simulink model "Modele_Eleve"  (R2021a)
settings: Solver=FixedStepAuto  StartTime=0.0  StopTime=10  FixedStep=2/1000  RelTol=1e-3
libraries: fl_lib x7, nesl_utility x3
settings Model: Creator=pt_ptsi  LastModifiedBy=xpess
settings SolverCC: AlgebraicLoopSolver=TrustRegion
settings DataIOCC: ReturnWorkspaceOutputs=off
settings DebuggingCC: SFMachineParentedDataDiag=warning  ArithmeticOperatorsInVariantConditions=warning
settings SFSimCC: SimUseLocalCustomCode=off  CustomCodeUndefinedFunction=UseInterfaceOnly
settings RTWCC: RTWUseLocalCustomCode=off
settings CodeAppCC: StateflowObjectComments=on
settings SimscapeCC: SimscapeNormalizeSystem=off

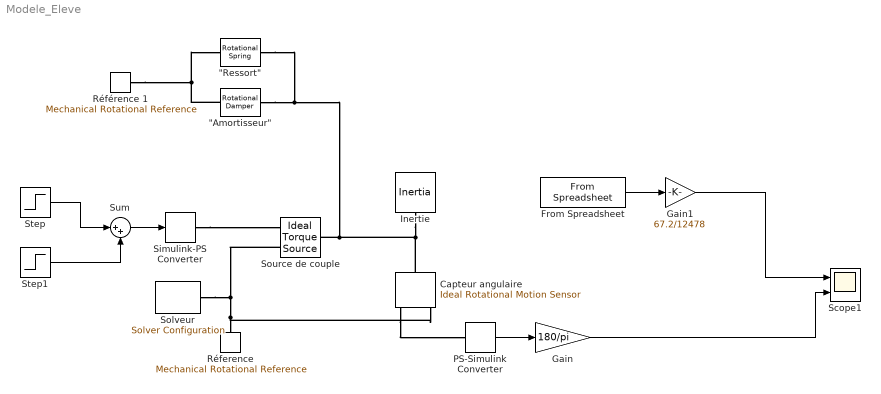
== system Modele_Eleve ==
  "\"Amortisseur\"" : fl_lib/Mechanical/Rotational Elements/Rotational Damper  D=0.01 N*m/(rad/s)  w_specify=off  w_priority=None  w=0 rad/s  w_nominal_specify=off  w_nominal_unit=rad/s  w_nominal_value=1  t_specify=off  t_priority=None  t=0 N*m  t_nominal_specify=off  t_nominal_unit=N*m  t_nominal_value=1
  "\"Ressort\"" : fl_lib/Mechanical/Rotational Elements/Rotational Spring  spr_rate=9.29 N*m/rad  w_specify=off  w_priority=None  w=0 rad/s  w_nominal_specify=off  w_nominal_unit=rad/s  w_nominal_value=1  t_specify=off  t_priority=None  t=0 N*m  t_nominal_specify=off  t_nominal_unit=N*m  t_nominal_value=1  phi_specify=off  phi_priority=High  phi=0 rad  phi_nominal_specify=off  phi_nominal_unit=rad  phi_nominal_value=1
  Capteur angulaire : fl_lib/Mechanical/Mechanical Sensors/Ideal Rotational Motion Sensor  wrap_angle=simscape.enum.onoff.off  offset=0 rad
  From Spreadsheet : FromSpreadsheet  FileName=C:\GitHub\PSI_Cy_04_ModelisationDynamique\TPs\TP_04_Drone\Essai\TestPendule.xlsx  SheetName=TestPendule  Range=A2:B502
  Gain : Gain  Gain=180/pi
  Gain1 : Gain  Gain=67.2/12478
  "Inertie " : fl_lib/Mechanical/Rotational Elements/Inertia  inertia=0.001 kg*m^2  num_ports=foundation.enum.numPorts2.one  w_specify=off  w_priority=High  w=0 rad/s  w_nominal_specify=off  w_nominal_unit=rad/s  w_nominal_value=1  t_specify=off  t_priority=None  t=0 N*m  t_nominal_specify=off  t_nominal_unit=N*m  t_nominal_value=1
  PS-Simulink Converter : nesl_utility/PS-Simulink Converter  PhysicalDomain=network_engine_domain  SubClassName=ps_output  LeftPortType=input  RightPortType=output  PseudoPeriodic=off  Frequencies=[]  Unit=1  AffineConversion=off
      settings: SourceProductBaseCode=PW,SS
  Réference : fl_lib/Mechanical/Rotational Elements/Mechanical Rotational Reference
  Référence 1 : fl_lib/Mechanical/Rotational Elements/Mechanical Rotational Reference
  Scope1 : Scope  NumInputPorts=2
  Simulink-PS Converter : nesl_utility/Simulink-PS Converter  PhysicalDomain=network_engine_domain  SubClassName=ps_input  LeftPortType=input  RightPortType=output  PseudoPeriodic=off  Frequencies=[]  NoiseDistribution=none  NoiseParameters=[]  Unit=1  AffineConversion=off  FilteringAndDerivatives=zero  SimscapeFilterOrder=1  InputFilterTimeConstant=0.001  UdotUserProvided=1
      settings: SourceProductBaseCode=PW,SS
  Solveur : nesl_utility/Solver Configuration  PhysicalDomain=network_engine_domain  SubClassName=solver  LeftPortType=input  RightPortType=generic  Tones=[]  Harmonics=[]  SimulateNoise=off  Profile=off  UseLocalSampling=off  EnableSwitchedLinearOptims=on  FrequencyDomain=off  UseCCode=off  RelTol=0.001  AbsTol=1e-06  MinStep=1e-09  ToWorkspace=off  RevertToSquareIcSolve=off  NumHomotopyIterations=100  PhasorMode=off  PhasorModeNumHarmonics=1  DoDC=off  ResidualTolerance=1e-09  UseLocalSolver=off  LocalSolverChoice=NE_BACKWARD_EULER_ADVANCER  LocalSolverSampleTime=0.001  DoFixedCost=off  MaxNonlinIter=3  MaxModeIter=2  ComputeImpulses=off  ImpulseIterations=2  LinearAlgebra=Sparse  EquationFormulation=NE_TIME_EF  DelaysMemoryBudget=1024  AutomaticFiltering=on  FilteringTimeConstant=0.001  PartitionStorageMethod=AS_NEEDED  PartitionMemoryBudget=1024  PartitionMethod=FAST
      settings: SourceProductBaseCode=PW,SS
  Source de couple : fl_lib/Mechanical/Mechanical Sources/Ideal Torque Source
  Step : Step  Time=0  After=0.6  SampleTime=0
  Step1 : Step  Time=10  After=-0.6  SampleTime=0
  Sum : Sum  Inputs=|++
  wires:
  Step/1 -> Sum/1
  Step1/1 -> Sum/2
  Sum/1 -> Simulink-PS Converter/1
  PS-Simulink Converter/1 -> Gain/1
  Gain/1 -> Scope1/2
  From Spreadsheet/1 -> Gain1/1
  Gain1/1 -> Scope1/1
  connections:
  Simulink-PS Converter/RConn1 -- Source de couple/RConn1
  "Inertie "/LConn1 -- "\"Ressort\""/RConn1 -- "\"Amortisseur\""/RConn1 -- Source de couple/LConn1 -- Capteur angulaire/LConn1
  Source de couple/RConn2 -- Solveur/RConn1 -- Capteur angulaire/RConn1 -- Réference/LConn1
  Capteur angulaire/RConn3 -- PS-Simulink Converter/LConn1
  Référence 1/LConn1 -- "\"Amortisseur\""/LConn1 -- "\"Ressort\""/LConn1
